simulink model "phase_estimator"  (R2024a)
settings: Solver=FixedStepAuto  StartTime=0.0  StopTime=Time  FixedStep=0.025  MaxStep=0.005  RelTol=1e-3
values from neighbouring files (symbols this model uses):
  time_sampl = 0.025    [main.m]
settings Model: Creator=totos  LastModifiedBy=marco

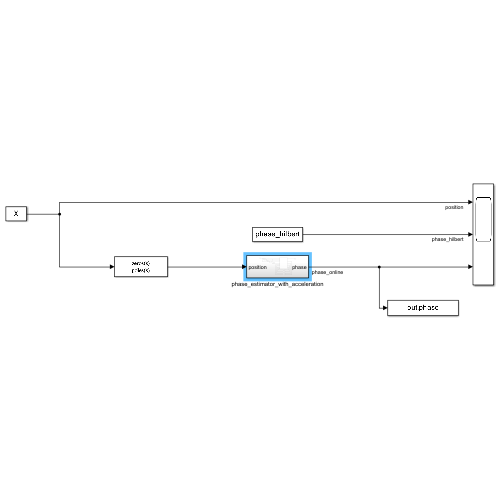
[thumbnail: Simulink's stored preview of the top-level diagram]
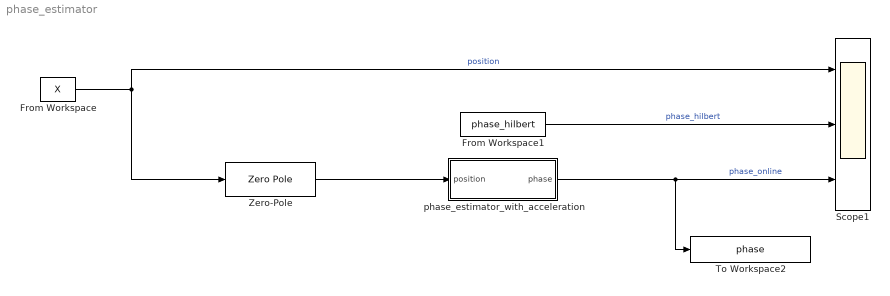
== system phase_estimator ==
  From Workspace : FromWorkspace  VariableName=X
  From Workspace1 : FromWorkspace  VariableName=phase_hilbert
  Scope1 : Scope  NumInputPorts=3
  To Workspace2 : ToWorkspace  VariableName=phase  SaveFormat=Timeseries  SampleTime=-1
  Zero-Pole : ZeroPole  Zeros=[]  Poles=[-1/time_sampl]  Gain=1/time_sampl
  phase_estimator_with_acceleration : Subsystem
  wires:
  From Workspace/1 -> Zero-Pole/1, Scope1/1  "position"
  From Workspace1/1 -> Scope1/2  "phase_hilbert"
  Zero-Pole/1 -> phase_estimator_with_acceleration/1(position)
  phase_estimator_with_acceleration/1(phase) -> To Workspace2/1, Scope1/3  "phase_online"

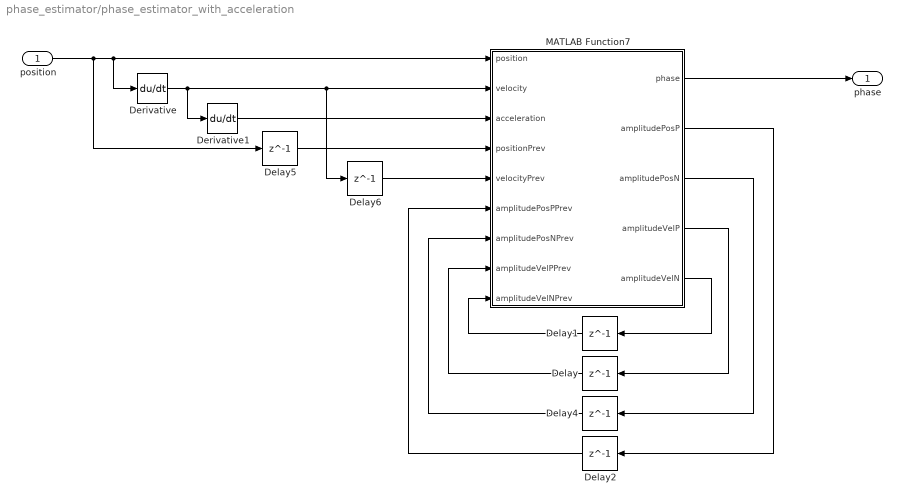
== system phase_estimator/phase_estimator_with_acceleration ==
  position : Inport
  Delay : Delay  DelayLength=1  InitialCondition=10
  Delay1 : Delay  DelayLength=1  InitialCondition=-10
  Delay2 : Delay  DelayLength=1  InitialCondition=5
  Delay4 : Delay  DelayLength=1  InitialCondition=-5
  Delay5 : Delay  DelayLength=1
  Delay6 : Delay  DelayLength=1
  Derivative : Derivative
  Derivative1 : Derivative
  MATLAB Function7 : MATLAB Function  TreatAsAtomicUnit=on
  phase : Outport
  wires:
  MATLAB Function7/1(phase) -> phase/1
  MATLAB Function7/2(amplitudePosP) -> Delay2/1
  position/1 -> MATLAB Function7/1(position), Derivative/1, Delay5/1
  Delay2/1 -> MATLAB Function7/6(amplitudePosPPrev)
  MATLAB Function7/4(amplitudeVelP) -> Delay/1
  MATLAB Function7/5(amplitudeVelN) -> Delay1/1
  MATLAB Function7/3(amplitudePosN) -> Delay4/1
  Delay1/1 -> MATLAB Function7/9(amplitudeVelNPrev)
  Delay4/1 -> MATLAB Function7/7(amplitudePosNPrev)
  Delay6/1 -> MATLAB Function7/5(velocityPrev)
  Delay5/1 -> MATLAB Function7/4(positionPrev)
  Derivative/1 -> MATLAB Function7/2(velocity), Delay6/1, Derivative1/1
  Delay/1 -> MATLAB Function7/8(amplitudeVelPPrev)
  Derivative1/1 -> MATLAB Function7/3(acceleration)

== matlab function phase_estimator/phase_estimator_with_acceleration/MATLAB Function7 ==
  data: position input; phase output; amplitudePosP output; amplitudePosN output; velocity input; acceleration input; positionPrev input; velocityPrev input; amplitudePosPPrev input; amplitudePosNPrev input; amplitudeVelPPrev input; amplitudeVelNPrev input; amplitudeVelP output; amplitudeVelN output
function [phase,amplitudePosP,amplitudePosN,amplitudeVelP,amplitudeVelN] = fcn(position,velocity,acceleration,positionPrev,velocityPrev,amplitudePosPPrev,amplitudePosNPrev,amplitudeVelPPrev,amplitudeVelNPrev)

if positionPrev < 0 && position >= 0 && velocity > 0
    amplitudeVelP = abs(velocity);
else
    amplitudeVelP = amplitudeVelPPrev;
end
		
if positionPrev >= 0 && position < 0 && velocity < 0
    amplitudeVelN = abs(velocity);
else
    amplitudeVelN = amplitudeVelNPrev;
end

if velocityPrev >= 0 && velocity < 0 && acceleration < 0
    amplitudePosP = abs(position);
else
    amplitudePosP = amplitudePosPPrev;
end
		
if velocityPrev < 0 && velocity >= 0 && acceleration > 0
    amplitudePosN = abs(position);
else
    amplitudePosN = amplitudePosNPrev;
end
		
		
if position >= 0
    positionNormalized = position / amplitudePosP;
else
    positionNormalized = position / amplitudePosN;
end
		
if velocity >= 0
    velocityNormalized = velocity / amplitudeVelP;
else
    velocityNormalized = velocity / amplitudeVelN;
end
phase = atan2(-velocityNormalized, positionNormalized);
